simulink model "mfsk"  (Simulink 6.4)
settings: Solver=FixedStepDiscrete  SolverMode=SingleTasking  StartTime=0.0  StopTime=inf  RelTol=1e-3
undefined symbols (not defined in the file or in its folder): Fs, get
libraries: commsink2 x2, commdigbbndcpm2 x2, commchan3 x1, commrandsrc2 x1, dspsnks4 x1
settings Model: Creator=ALEX  LastModifiedBy=student
settings OptimizationCC: InitFltsAndDblsToZero=off
settings DebuggingCC: SignalResolutionControl=UseLocalSettings  MultiTaskDSMMsg=error  MultiTaskCondExecSysMsg=error
settings GRTTargetCC: TargetFcnLib=ansi_tfl_table_tmw.mat

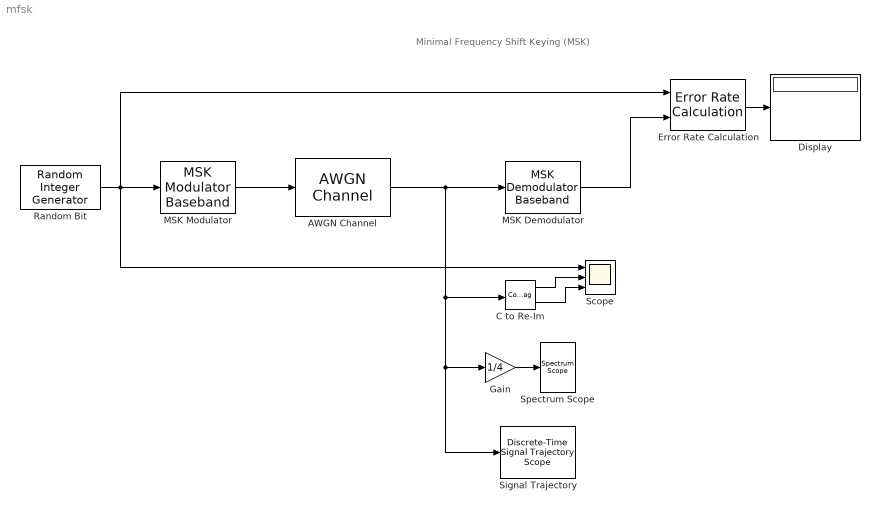
== system mfsk ==
  note: Minimal Frequency Shift Keying (MSK)
  AWGN Channel : commchan3/AWGN Channel  SystemSampleTime=-1  seed=67  noiseMode="Signal to noise ratio  (Es/No)"  EbNodB=3  EsNodB=100  SNRdB=10  bitsPerSym=1  Ps=1  Tsym=1  variance=0
  C to Re-Im : ComplexToRealImag
  Display : Display
  Error Rate Calculation : commsink2/Error Rate Calculation  N=9  st_delay=0  cp_mode=Entire frame  subframe=[]  PMode=Port  WsName=ErrorVec  RsMode2=off  stop=off  numErr=1000  maxBits=100000
  Gain : Gain  Gain=1/4  ParameterDataType=fixdt(1, 16)  OutDataType=fixdt(1, 16)
  MSK Demodulator : commdigbbndcpm2/MSK Demodulator Baseband  SystemSampleTime=-1  outputType=Bit  phaseOffset=0  samplesPerSymbol=16  traceBack=8  outDType=boolean
  MSK Modulator : commdigbbndcpm2/MSK Modulator Baseband  SystemSampleTime=-1  inputType=Bit  phaseOffset=0  samplesPerSymbol=16  outDataType=double
  Random Bit : commrandsrc2/Random Integer Generator  SystemSampleTime=-1  mul=2  seed=37  Ts=1  frameBased=off  sampPerFrame=8  orient=off  outDataType=boolean
  Scope : Scope  NumInputPorts=3
      settings: TimeRange=10  YMin=0~-1.25~-1.25  YMax=1.2~1.25~1.25
  Signal Trajectory : commsink2/Discrete-Time Signal Trajectory Scope  Tag=SignalTrajectory  SystemSampleTime=-1  sampPerSymb=8  offsetEye=0  numTraces=40  numNewFrames=10  LineStyles=-  LineColors=b  fading=on  render=on  AxisGrid=on  xMin=-3.3  xMax=3.315  yMin=-3.3  yMax=3.315  inphaseLabel=In-phase Amplitude  quadratureLabel=Quadrature Amplitude  openScopeAtSimStart=off  FrameNumber=off  FigPos=[360 435 560 487]  figTitle=Signal Trajectory  numLinesMax=8  block_type_=xy
  Spectrum Scope : dspsnks4/Spectrum Scope  DialogController=dspdialog.SpectrumScope  DialogControllerArgs=DataTag0  SystemSampleTime=-1  ScopeProperties=on  Domain=Frequency  HorizSpan=1  UseBuffer=on  BufferSize=2048  Overlap=0  inpFftLenInherit=off  FFTlength=4096  numAvg=50  DisplayProperties=off  AxisGrid=on  Memory=off  FrameNumber=on  AxisLegend=off  AxisZoom=off  OpenScopeAtSimStart=on  OpenScopeImmediately=off  FigPos=get(0,'defaultfigureposition')  AxisProperties=off  XUnits=Hertz  XRange=[-Fs/2...Fs/2]  InheritXIncr=on  XIncr=1.0  XLabel=Samples  YUnits=dB  YLabel=Magnitude-squared, dB  LineProperties=off  wintypeSpecScope=Hamming  RsSpecScope=50  betaSpecScope=5  winsampSpecScope=Symmetric
      settings: YMin=-69.6891932040416  YMax=6.57958785526319
  wires:
  Error Rate Calculation/1 -> Display/1
  AWGN Channel/1 -> MSK Demodulator/1, C to Re-Im/1, Signal Trajectory/1, Gain/1
  Random Bit/1 -> MSK Modulator/1, Error Rate Calculation/1, Scope/1
  MSK Modulator/1 -> AWGN Channel/1
  MSK Demodulator/1 -> Error Rate Calculation/2
  Gain/1 -> Spectrum Scope/1
  C to Re-Im/1 -> Scope/2
  C to Re-Im/2 -> Scope/3
